simulink model "gm_BlobAnalysisHDL"  (R2022b)
settings: Solver=FixedStepDiscrete  StartTime=0.0  StopTime=1/60  RelTol=1e-3
PreLoadFcn:
  | model_init_cca
InitFcn:
  | model_init_cca
undefined symbols (not defined in the file or in its folder): closenhood, gray, MaxBlobs, numCols, numRows, Rec, rgbmap24, SDTV, Ts
libraries: hdlsllib x37, simulink x21, hdlmdlgenlib x7, visionhdlutilities x5, visionhdlio x2, visiontextngfix x2, visionhdlmorphops x1, visionhdlconversions x1, visionsources x1, visiongeotforms x1
(part 2 of 3)

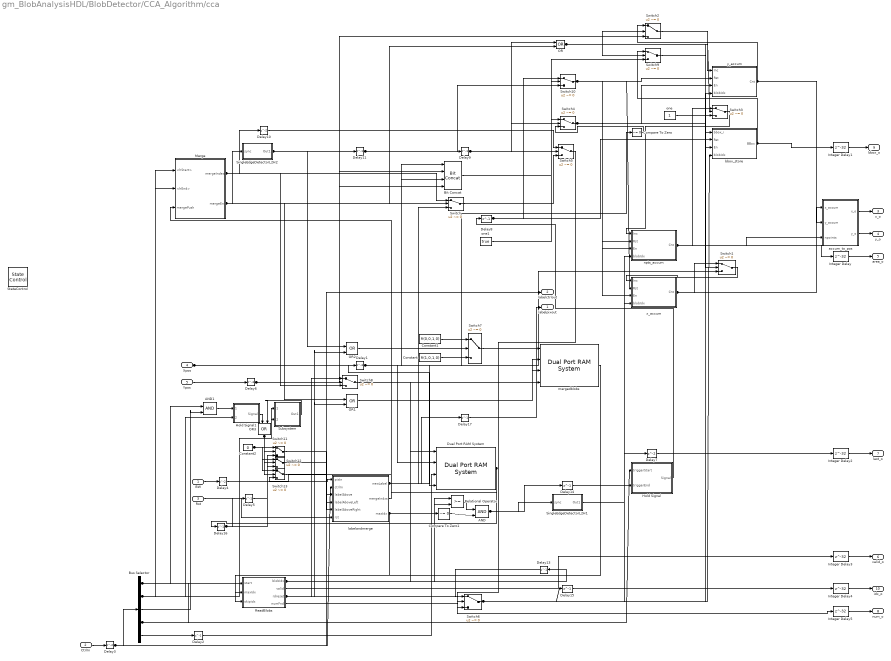
== system gm_BlobAnalysisHDL/BlobDetector/CCA_Algorithm/cca ==
  BW : Inport  OutDataTypeStr=boolean  PortDimensions=1  SampleTime=1.2796101795549e-07
  CtrlIn : Inport  Port=2
  Rst : Inport  Port=3  OutDataTypeStr=boolean  PortDimensions=1  SampleTime=1.2796101795549e-07
  Xpos : Inport  Port=4  OutDataTypeStr=fixdt(0, 9, 0)  PortDimensions=1  SampleTime=1.2796101795549e-07
  Ypos : Inport  Port=5  OutDataTypeStr=uint8  PortDimensions=1  SampleTime=1.2796101795549e-07
  AND : Logic  IconShape=distinctive  AllPortsSameDT=off  OutDataTypeStr=boolean
  AND1 : Logic  IconShape=distinctive  AllPortsSameDT=off  OutDataTypeStr=boolean
  Bit Concat : hdlsllib/Logic and Bit Operations/Bit Concat  numInputs=4
  Bus Selector : BusSelector  OutputSignals=hStart,hEnd,vStart,vEnd,valid
  Compare To Zero : simulink/Logic and Bit Operations/Compare To Zero  relop=~=  OutDataTypeStr=boolean
  Compare To Zero1 : simulink/Logic and Bit Operations/Compare To Zero  relop=~=  OutDataTypeStr=boolean
  Constant : Constant  Value=fi(1,0,1,0)  SampleTime=-1
  Constant1 : Constant  Value=fi(0,0,1,0)  SampleTime=-1
  Constant2 : Constant  Value=0  OutDataTypeStr=fixdt(0,ceil(log2(MaxBlobs)),0)  SampleTime=-1
  Delay1 : Delay  DelayLength=3
  Delay10 : Delay
  Delay{2,5,9,11,13,16..17} (7 alike) : Delay  DelayLength=1
  Delay14 : Delay  DelayLength=1  InitialCondition=0
  Delay15 : Delay  DelayLength=1  InitialCondition=0
  Delay3 : Delay
  Delay4 : Delay
  Delay6 : Delay  DelayLength=3
  Delay7 : Delay  InitialCondition=0
  Delay8 : Delay  DelayLength=1  InitialCondition=0
  Dual Port RAM System : hdlsllib/HDL RAMs/Dual Port RAM System  RAMType=Simple dual port  WriteOutputValue=Old data  RAMInitialValue=0  SimulateUsing=Code generation
  Hold Signal : Subsystem
  Hold Signal1 : Subsystem
  Integer Delay{,1..5} (6 alike) : Delay  DelayLength=32  InitialCondition=0
  Merge : Subsystem
  OR{,1..3} (4 alike) : Logic  Operator=OR  IconShape=distinctive  AllPortsSameDT=off  OutDataTypeStr=boolean
  ReadBlobs : Subsystem
  Relational Operator : RelationalOperator  OutDataTypeStr=boolean  RndMeth=Simplest  InputSameDT=off
  SingleEdgeDetectorL2H1 : Subsystem
  SingleEdgeDetectorL2H2 : Subsystem
  StateControl : StateControl  StateControl=Synchronous
  Subsystem : Subsystem
  Switch{,1..13} (14 alike) : Switch  Criteria=u2 ~= 0  SaturateOnIntegerOverflow=off  InputSameDT=off
  accum_to_pos : Subsystem
  bbox_store : Subsystem  mask(Accumulator){MaxVal=double(76800)}
      mask prompts: MaxVal "Accumulator Maximum Value"
      mask help: Accumulate values
  labelandmerge : Subsystem
  mergedblobs : hdlsllib/HDL RAMs/Dual Port RAM System  RAMType=Simple dual port  WriteOutputValue=Old data  RAMInitialValue=0  SimulateUsing=Code generation
  npts_accum : Subsystem  mask(Accumulator){MaxVal=double(76800)}
      mask prompts: MaxVal "Accumulator Maximum Value"
      mask help: Accumulate values
  one : Constant  OutDataTypeStr=Inherit: Inherit via back propagation  SampleTime=-1
  one1 : Constant  Value=true  OutDataTypeStr=Inherit: Inherit via back propagation  SampleTime=-1
  x_accum : Subsystem  mask(Accumulator){MaxVal=double(12326400)}
      mask prompts: MaxVal "Accumulator Maximum Value"
      mask help: Accumulate values
  y_accum : Subsystem  mask(Accumulator){MaxVal=double(9254400)}
      mask prompts: MaxVal "Accumulator Maximum Value"
      mask help: Accumulate values
  labelpixout : Outport  SampleTime=1.2796101795549e-07  VectorParamsAs1DForOutWhenUnconnected=off
  labelctrlout : Outport  Port=2  VectorParamsAs1DForOutWhenUnconnected=off
  x_o : Outport  Port=3  SampleTime=1.2796101795549e-07  VectorParamsAs1DForOutWhenUnconnected=off
  y_o : Outport  Port=4  SampleTime=1.2796101795549e-07  VectorParamsAs1DForOutWhenUnconnected=off
  area_o : Outport  Port=5  SampleTime=1.2796101795549e-07  VectorParamsAs1DForOutWhenUnconnected=off
  valid_o : Outport  Port=6  SampleTime=1.2796101795549e-07  VectorParamsAs1DForOutWhenUnconnected=off
  last_o : Outport  Port=7  SampleTime=1.2796101795549e-07  VectorParamsAs1DForOutWhenUnconnected=off
  num_o : Outport  Port=8  SampleTime=1.2796101795549e-07  VectorParamsAs1DForOutWhenUnconnected=off
  bbox_o : Outport  Port=9  SampleTime=1.2796101795549e-07  VectorParamsAs1DForOutWhenUnconnected=off
  idx_o : Outport  Port=10  SampleTime=1.2796101795549e-07  VectorParamsAs1DForOutWhenUnconnected=off
  wires:
  AND/1 -> Delay14/1, SingleEdgeDetectorL2H1/1(sync)
  AND1/1 -> Hold Signal1/1(triggerStart)
  Bit Concat/1 -> Switch9/3
  Bus Selector/1 -> AND1/1, Subsystem/1(<hStart>), Merge/1(<hStart>)
  Bus Selector/2 -> Subsystem/2(<hEnd>), Hold Signal1/2(triggerEnd), Merge/2(<hEnd>)
  Bus Selector/3 -> AND1/2
  Bus Selector/4 -> Hold Signal/1(triggerStart), ReadBlobs/1(start)
  Bus Selector/5 -> Delay2/1
  Compare To Zero/1 -> Switch4/3
  Compare To Zero1/1 -> AND/2
  Constant/1 -> Switch7/3
  Constant1/1 -> Switch7/1
  Constant2/1 -> Switch13/1, Switch12/1, Switch11/1
  Delay1/1 -> Bit Concat/3, Bit Concat/1, Switch1/3, Dual Port RAM System/2
  Delay10/1 -> Switch5/1
  Delay11/1 -> Switch10/3, Delay9/1
  Delay13/1 -> Switch6/1
  Delay14/1 -> Hold Signal/2(triggerEnd)
  Delay15/1 -> Integer Delay4/1
  Delay17/1 -> labelpixout/1
  Delay2/1 -> Dual Port RAM System/3
  Delay3/1 -> Bus Selector/1, labelctrlout/1, labelandmerge/2(ctrlIn)
  Delay4/1 -> labelandmerge/1(pixIn)
  Delay6/1 -> Bit Concat/4, Bit Concat/2, Switch2/3
  Delay7/1 -> Integer Delay2/1
  Delay8/1 -> Switch10/2, Switch10/1, bbox_store/2(Rst)
  Delay9/1 -> Switch5/2, Switch4/2, OR/1
  Hold Signal/1(Signal) -> Delay8/1
  Hold Signal1/1(Signal) -> OR3/1
  Integer Delay/1 -> area_o/1
  Integer Delay1/1 -> bbox_o/1
  Integer Delay2/1 -> last_o/1
  Integer Delay3/1 -> valid_o/1
  Integer Delay4/1 -> idx_o/1
  Integer Delay5/1 -> num_o/1
  Merge/1(mergeIndex) -> Switch/1, Delay10/1, Switch8/3
  Merge/2(mergeEn) -> Switch/2, OR/2, SingleEdgeDetectorL2H2/1(sync), OR1/1
  OR/1 -> Switch9/2, Switch1/2, Switch2/2, Switch3/2
  OR3/1 -> Switch13/2, Switch12/2, Switch11/2
  ReadBlobs/1(blobIdx) -> Relational Operator/1, Delay13/1, Switch8/1, mergedblobs/4
  ReadBlobs/2(valid) -> Integer Delay3/1
  ReadBlobs/3(rdreset) -> Switch6/2, Switch8/2, OR2/2, OR1/2
  ReadBlobs/4(numFnd) -> Integer Delay5/1
  Relational Operator/1 -> AND/1
  SingleEdgeDetectorL2H1/1(Out1) -> Delay7/1
  SingleEdgeDetectorL2H2/1(Out1) -> Delay11/1, OR2/1
  Subsystem/1(Out1) -> OR3/2
  Switch/1 -> Switch5/3
  Switch10/1 -> x_accum/2(Rst), y_accum/2(Rst), npts_accum/2(Rst)
  Switch4/1 -> bbox_store/3(En), x_accum/3(En), y_accum/3(En), npts_accum/3(En)
  Switch5/1 -> Switch6/3
  Switch6/1 -> Delay15/1, bbox_store/4(blobIdx), x_accum/4(blobIdx), y_accum/4(blobIdx), npts_accum/4(blobIdx)
  accum_to_pos/1(x_o) -> x_o/1
  accum_to_pos/2(y_o) -> y_o/1
  bbox_store/1(BBox) -> Integer Delay1/1, Switch9/1
  labelandmerge/1(newLabel) -> Switch/3, Compare To Zero/1, Delay17/1, Dual Port RAM System/1
  labelandmerge/2(mergeIndxs) -> Merge/3(mergePush)
  labelandmerge/3(maxIdx) -> Relational Operator/2, Compare To Zero1/1, ReadBlobs/2(maxIdx)
  npts_accum/1(Cnt) -> Integer Delay/1, accum_to_pos/3(npoints), Switch3/1
  one/1 -> Switch3/3
  one1/1 -> Switch4/1
  x_accum/1(Cnt) -> accum_to_pos/1(x_accum), Switch1/1
  y_accum/1(Cnt) -> accum_to_pos/2(y_accum), Switch2/1
  BW/1 -> Delay4/1
  CtrlIn/1 -> Delay3/1
  Rst/1 -> labelandmerge/6(rst)
  Xpos/1 -> Delay1/1, Dual Port RAM System/4
  Ypos/1 -> Delay6/1
  Switch9/1 -> bbox_store/1(bbox_i)
  Switch13/1 -> labelandmerge/5(labelAboveRight)
  Switch12/1 -> labelandmerge/4(labelAboveLeft)
  Delay5/1 -> Switch12/3
  Switch11/1 -> labelandmerge/3(labelAbove)
  Dual Port RAM System/1 -> Switch13/3, Delay16/1
  Delay16/1 -> Switch11/3, Delay5/1
  OR1/1 -> mergedblobs/3
  Switch8/1 -> mergedblobs/2
  Switch7/1 -> mergedblobs/1
  OR2/1 -> Switch7/2
  mergedblobs/1 -> ReadBlobs/3(skipidx)
  Switch1/1 -> x_accum/1(Inc)
  Switch2/1 -> y_accum/1(Inc)
  Switch3/1 -> npts_accum/1(Inc)

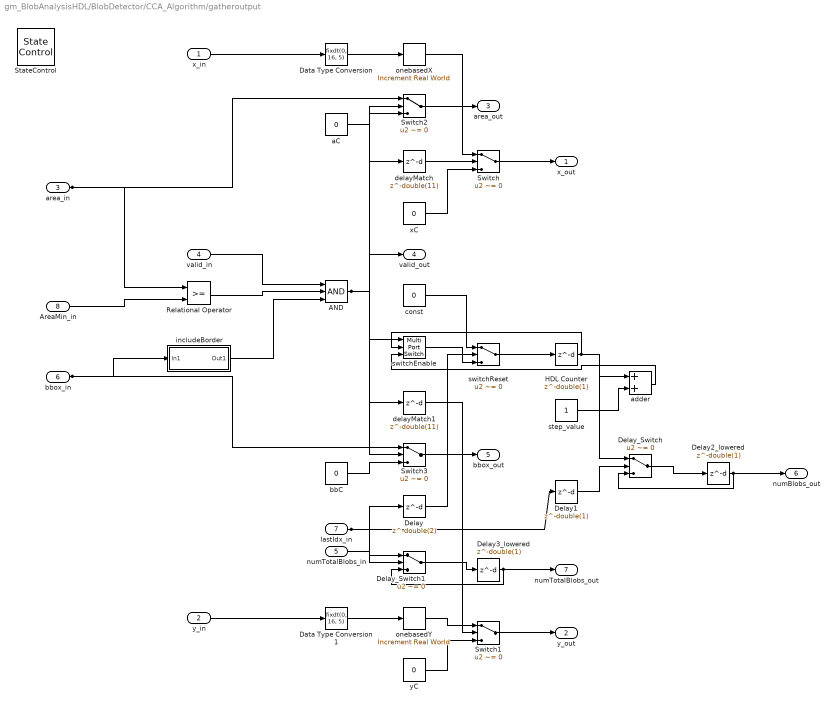
== system gm_BlobAnalysisHDL/BlobDetector/CCA_Algorithm/gatheroutput ==
  x_in : Inport  OutDataTypeStr=fixdt(0, 56, 30)  PortDimensions=1  SampleTime=1.2796101795549e-07
  y_in : Inport  Port=2  OutDataTypeStr=fixdt(0, 56, 30)  PortDimensions=1  SampleTime=1.2796101795549e-07
  area_in : Inport  Port=3  OutDataTypeStr=fixdt(0, 17, 0)  PortDimensions=1  SampleTime=1.2796101795549e-07
  valid_in : Inport  Port=4  OutDataTypeStr=boolean  PortDimensions=1  SampleTime=1.2796101795549e-07
  numTotalBlobs_in : Inport  Port=5  OutDataTypeStr=uint16  PortDimensions=1  SampleTime=1.2796101795549e-07
  bbox_in : Inport  Port=6  OutDataTypeStr=fixdt(0, 34, 0)  PortDimensions=1  SampleTime=1.2796101795549e-07
  lastIdx_in : Inport  Port=7  OutDataTypeStr=boolean  PortDimensions=1  SampleTime=1.2796101795549e-07
  AreaMin_in : Inport  Port=8  OutDataTypeStr=uint32  PortDimensions=1  SampleTime=1.2796101795549e-07
  AND : Logic  Inputs=3  AllPortsSameDT=off  OutDataTypeStr=boolean  SampleTime=1.2796101795549e-07
  Data Type Conversion : DataTypeConversion  OutDataTypeStr=fixdt(0, 16, 5)  SampleTime=1.2796101795549e-07  SaturateOnIntegerOverflow=off  RndMeth=Floor
  Data Type Conversion1 : DataTypeConversion  OutDataTypeStr=fixdt(0, 16, 5)  SampleTime=1.2796101795549e-07  SaturateOnIntegerOverflow=off  RndMeth=Floor
  Delay : Delay  DelayLength=double(2)  InitialCondition=1  SampleTime=1.2796101795549e-07
  Delay1 : Delay  DelayLength=double(1)  InitialCondition=1  SampleTime=1.2796101795549e-07
  Delay2_lowered : Delay  DelayLength=double(1)  InitialCondition=0  SampleTime=1.2796101795549e-07
  Delay3_lowered : Delay  DelayLength=double(1)  InitialCondition=0  SampleTime=1.2796101795549e-07
  Delay_Switch : Switch  Criteria=u2 ~= 0  Threshold=double(0)  OutDataTypeStr=uint16  SampleTime=1.2796101795549e-07  SaturateOnIntegerOverflow=off  InputSameDT=off
  Delay_Switch1 : Switch  Criteria=u2 ~= 0  Threshold=double(0)  OutDataTypeStr=uint16  SampleTime=1.2796101795549e-07  SaturateOnIntegerOverflow=off  InputSameDT=off
  HDL Counter : Delay  DelayLength=double(1)  InitialCondition=0  SampleTime=1.2796101795549e-07
  Relational Operator : RelationalOperator  OutDataTypeStr=boolean  SampleTime=1.2796101795549e-07  InputSameDT=off
  StateControl : StateControl  StateControl=Synchronous
  Switch : Switch  Criteria=u2 ~= 0  Threshold=double(0)  OutDataTypeStr=fixdt(0, 16, 5)  SampleTime=1.2796101795549e-07  SaturateOnIntegerOverflow=off  InputSameDT=off
  Switch1 : Switch  Criteria=u2 ~= 0  Threshold=double(0)  OutDataTypeStr=fixdt(0, 16, 5)  SampleTime=1.2796101795549e-07  SaturateOnIntegerOverflow=off  InputSameDT=off
  Switch2 : Switch  Criteria=u2 ~= 0  Threshold=double(0)  OutDataTypeStr=fixdt(0, 17, 0)  SampleTime=1.2796101795549e-07  SaturateOnIntegerOverflow=off  InputSameDT=off
  Switch3 : Switch  Criteria=u2 ~= 0  Threshold=double(0)  OutDataTypeStr=fixdt(0, 34, 0)  SampleTime=1.2796101795549e-07  SaturateOnIntegerOverflow=off  InputSameDT=off
  aC : Constant  Value=0  OutDataTypeStr=fixdt(0, 17, 0)  SampleTime=1.2796101795549e-07
  adder : Sum  AccumDataTypeStr=uint16  OutDataTypeStr=uint16  SampleTime=1.2796101795549e-07
  bbC : Constant  Value=0  OutDataTypeStr=fixdt(0, 34, 0)  SampleTime=1.2796101795549e-07
  const : Constant  Value=0  VectorParams1D=off  OutDataTypeStr=uint16  SampleTime=1.2796101795549e-07
  delayMatch : Delay  DelayLength=double(11)  InitialCondition=0  SampleTime=1.2796101795549e-07
  delayMatch1 : Delay  DelayLength=double(11)  InitialCondition=0  SampleTime=1.2796101795549e-07
  includeBorder : Subsystem
  onebasedX : simulink/Additional Math & Discrete/Additional Math: Increment - Decrement/Increment Real World
  onebasedY : simulink/Additional Math & Discrete/Additional Math: Increment - Decrement/Increment Real World
  step_value : Constant  VectorParams1D=off  OutDataTypeStr=uint16  SampleTime=1.2796101795549e-07
  switchEnable : MultiPortSwitch  DataPortOrder=Zero-based contiguous  Inputs=2  DiagnosticForDefault=None  zeroidx=on  OutDataTypeStr=uint16  SampleTime=1.2796101795549e-07  SaturateOnIntegerOverflow=off  InputSameDT=off
  switchReset : Switch  Criteria=u2 ~= 0  Threshold=double(0)  OutDataTypeStr=uint16  SampleTime=1.2796101795549e-07  SaturateOnIntegerOverflow=off  InputSameDT=off
  xC : Constant  Value=0  OutDataTypeStr=fixdt(0, 16, 5)  SampleTime=1.2796101795549e-07
  yC : Constant  Value=0  OutDataTypeStr=fixdt(0, 16, 5)  SampleTime=1.2796101795549e-07
  x_out : Outport  SampleTime=1.2796101795549e-07  VectorParamsAs1DForOutWhenUnconnected=off
  y_out : Outport  Port=2  SampleTime=1.2796101795549e-07  VectorParamsAs1DForOutWhenUnconnected=off
  area_out : Outport  Port=3  SampleTime=1.2796101795549e-07  VectorParamsAs1DForOutWhenUnconnected=off
  valid_out : Outport  Port=4  SampleTime=1.2796101795549e-07  VectorParamsAs1DForOutWhenUnconnected=off
  bbox_out : Outport  Port=5  SampleTime=1.2796101795549e-07  VectorParamsAs1DForOutWhenUnconnected=off
  numBlobs_out : Outport  Port=6  SampleTime=1.2796101795549e-07  VectorParamsAs1DForOutWhenUnconnected=off
  numTotalBlobs_out : Outport  Port=7  SampleTime=1.2796101795549e-07  VectorParamsAs1DForOutWhenUnconnected=off
  wires:
  delayMatch/1 -> Switch/2
  Data Type Conversion/1 -> onebasedX/1
  Data Type Conversion1/1 -> onebasedY/1
  Delay/1 -> switchReset/2
  Delay1/1 -> Delay_Switch/2
  Delay2_lowered/1 -> numBlobs_out/1, Delay_Switch/3
  Delay3_lowered/1 -> numTotalBlobs_out/1, Delay_Switch1/3
  Relational Operator/1 -> AND/2
  Switch/1 -> x_out/1
  Switch1/1 -> y_out/1
  Switch2/1 -> area_out/1
  Switch3/1 -> bbox_out/1
  aC/1 -> Switch2/3
  bbC/1 -> Switch3/3
  includeBorder/1(Out1) -> AND/3
  onebasedX/1 -> Switch/1
  onebasedY/1 -> Switch1/1
  xC/1 -> Switch/3
  yC/1 -> Switch1/3
  HDL Counter/1 -> switchEnable/2, adder/1, Delay_Switch/1
  const/1 -> switchReset/1
  step_value/1 -> adder/2
  x_in/1 -> Data Type Conversion/1
  y_in/1 -> Data Type Conversion1/1
  area_in/1 -> Switch2/1, Relational Operator/1
  valid_in/1 -> AND/1
  numTotalBlobs_in/1 -> Delay_Switch1/1
  bbox_in/1 -> Switch3/1, includeBorder/1(In1)
  lastIdx_in/1 -> Delay1/1, Delay/1, Delay_Switch1/2
  AreaMin_in/1 -> Relational Operator/2
  delayMatch1/1 -> Switch1/2
  AND/1 -> delayMatch1/1, delayMatch/1, Switch3/2, Switch2/2, valid_out/1, switchEnable/1
  Delay_Switch1/1 -> Delay3_lowered/1
  adder/1 -> switchEnable/3
  switchEnable/1 -> switchReset/3
  switchReset/1 -> HDL Counter/1
  Delay_Switch/1 -> Delay2_lowered/1

== system gm_BlobAnalysisHDL/BlobDetector/CacheResultForXfer/splitBBox ==
  In1 : Inport  OutDataTypeStr=fixdt(0, 34, 0)  PortDimensions=1  SampleTime=1.2796101795549e-07
  Bit Slice4 : hdlsllib/Logic and Bit Operations/Bit Slice  lidx=ceil(log2(numRows))-1  ridx=0
  Bit Slice5 : hdlsllib/Logic and Bit Operations/Bit Slice  lidx=ceil(log2(numRows))+ceil(log2(numCols))-1  ridx=ceil(log2(numRows))
  Bit Slice6 : hdlsllib/Logic and Bit Operations/Bit Slice  lidx=2*ceil(log2(numRows))+ceil(log2(numCols))-1  ridx=ceil(log2(numRows))+ceil(log2(numCols))
  Bit Slice7 : hdlsllib/Logic and Bit Operations/Bit Slice  lidx=2*ceil(log2(numRows))+2*ceil(log2(numCols))-1  ridx=2*ceil(log2(numRows))+ceil(log2(numCols))
  X1 : Outport  SampleTime=1.2796101795549e-07  VectorParamsAs1DForOutWhenUnconnected=off
  Y1 : Outport  Port=2  SampleTime=1.2796101795549e-07  VectorParamsAs1DForOutWhenUnconnected=off
  X2 : Outport  Port=3  SampleTime=1.2796101795549e-07  VectorParamsAs1DForOutWhenUnconnected=off
  Y2 : Outport  Port=4  SampleTime=1.2796101795549e-07  VectorParamsAs1DForOutWhenUnconnected=off
  wires:
  Bit Slice4/1 -> Y2/1
  Bit Slice5/1 -> X2/1
  Bit Slice6/1 -> Y1/1
  Bit Slice7/1 -> X1/1
  In1/1 -> Bit Slice7/1, Bit Slice6/1, Bit Slice5/1, Bit Slice4/1

== system gm_BlobAnalysisHDL/BlobDetector/CCA_Algorithm/PaletteMap/bit2RGB ==
  In1 : Inport  OutDataTypeStr=fixdt(0, 24, 0)  PortDimensions=1  SampleTime=1.2796101795549e-07
  Blue : simulink/Logic and Bit Operations/Extract Bits  bitsToExtract=Range of bits  numBits=8  bitIdxRange=[0 7]  outScalingMode=Treat bit field as an integer
  Green : simulink/Logic and Bit Operations/Extract Bits  bitsToExtract=Range of bits  numBits=8  bitIdxRange=[8 15]  outScalingMode=Treat bit field as an integer
  Red : simulink/Logic and Bit Operations/Extract Bits  bitsToExtract=Range of bits  numBits=8  bitIdxRange=[16 23]  outScalingMode=Treat bit field as an integer
  Vector Concatenate : Concatenate  NumInputs=3  Mode=Multidimensional array  ConcatenateDimension=2
  Out1 : Outport  SampleTime=1.2796101795549e-07  VectorParamsAs1DForOutWhenUnconnected=off
  wires:
  Blue/1 -> Vector Concatenate/3
  Green/1 -> Vector Concatenate/2
  Red/1 -> Vector Concatenate/1
  Vector Concatenate/1 -> Out1/1
  In1/1 -> Red/1, Green/1, Blue/1

== system gm_BlobAnalysisHDL/BlobDetector/CCA_Algorithm/Pixel Stream FIFO/CastIfBoolean ==
  u : Inport  OutDataTypeStr=uint8  PortDimensions=1  SampleTime=1.2796101795549e-07
  visionhdlutilities_c1_CastIfBoolean : MATLAB Function  TreatAsAtomicUnit=on
      settings: LibrarySourceBlock=visionhdlutilities/Pixel Stream FIFO/CastIfBoolean
  y : Outport  SampleTime=1.2796101795549e-07  VectorParamsAs1DForOutWhenUnconnected=off
  wires:
  visionhdlutilities_c1_CastIfBoolean/1(y) -> y/1
  u/1 -> visionhdlutilities_c1_CastIfBoolean/1(u)

== system gm_BlobAnalysisHDL/BlobDetector/CCA_Algorithm/Pixel Stream FIFO/Input Control Validation  ==
  ctrlIn : Inport
  ControlBalance{,1..6} (7 alike) : Delay  DelayLength=1
  InLineInFrameTest : Subsystem
  Logical Operator{1..6} (6 alike) : Logic  AllPortsSameDT=off  OutDataTypeStr=boolean
  Logical Operator7 : Logic  Operator=OR  AllPortsSameDT=off  OutDataTypeStr=boolean
  Logical Operator8 : Logic  Operator=OR  AllPortsSameDT=off  OutDataTypeStr=boolean
  Pixel Control Bus Creator : visionhdlutilities/Pixel Control Bus Creator
  Pixel Control Bus Selector : BusSelector  OutputSignals=hStart,hEnd,vStart,vEnd,valid
  ctrlOut : Outport  VectorParamsAs1DForOutWhenUnconnected=off
  wires:
  ControlBalance/1 -> Pixel Control Bus Selector/1
  ControlBalance1/1 -> Logical Operator5/1
  ControlBalance2/1 -> Logical Operator6/1, Logical Operator5/2
  ControlBalance3/1 -> Logical Operator3/1
  ControlBalance4/1 -> Logical Operator2/1
  ControlBalance5/1 -> Pixel Control Bus Creator/2
  ControlBalance6/1 -> Pixel Control Bus Creator/4
  InLineInFrameTest/1(InLineInFrame) -> Logical Operator6/2, Logical Operator4/2, Logical Operator3/2, Logical Operator2/2, Logical Operator1/2, ControlBalance1/1
  Logical Operator1/1 -> Logical Operator8/1
  Logical Operator2/1 -> Pixel Control Bus Creator/3
  Logical Operator3/1 -> Pixel Control Bus Creator/1
  Logical Operator4/1 -> Logical Operator8/2, ControlBalance6/1
  Logical Operator5/1 -> Logical Operator7/2
  Logical Operator6/1 -> Logical Operator7/1
  Logical Operator7/1 -> Pixel Control Bus Creator/5
  Logical Operator8/1 -> ControlBalance5/1
  Pixel Control Bus Creator/1 -> ctrlOut/1
  Pixel Control Bus Selector/1 -> ControlBalance3/1
  Pixel Control Bus Selector/2 -> Logical Operator1/1
  Pixel Control Bus Selector/3 -> ControlBalance4/1
  Pixel Control Bus Selector/4 -> Logical Operator4/1
  Pixel Control Bus Selector/5 -> ControlBalance2/1
  ctrlIn/1 -> ControlBalance/1, InLineInFrameTest/1(ctrlIn)

== system gm_BlobAnalysisHDL/BlobDetector/CCA_Algorithm/Pixel Stream FIFO/InputSizeValidation ==
  pixelIn : Inport  OutDataTypeStr=uint8  PortDimensions=1  SampleTime=1.2796101795549e-07
  ctrlIn : Inport  Port=2
  noHDL : visionhdlutilities/Pixel Stream FIFO/InputSizeValidation/noHDL  SystemSampleTime=-1  VariantActivationTime=update diagram  Latency=0  AutoFrameSizeCalculation=off
  wires:
  pixelIn/1 -> noHDL/1
  ctrlIn/1 -> noHDL/2

== system gm_BlobAnalysisHDL/BlobDetector/CCA_Algorithm/Pixel Stream FIFO/Memory Controller ==
  hEnd : Inport  OutDataTypeStr=boolean  PortDimensions=1  SampleTime=1.2796101795549e-07
  readCountIn : Inport  Port=2  OutDataTypeStr=fixdt(0, 11, 0)  PortDimensions=1  SampleTime=1.2796101795549e-07
  writeCountLimit : Inport  Port=3  OutDataTypeStr=fixdt(0, 11, 0)  PortDimensions=1  SampleTime=1.2796101795549e-07
  vStart : Inport  Port=4  OutDataTypeStr=boolean  PortDimensions=1  SampleTime=1.2796101795549e-07
  visionhdlutilities_c2_Memory_Controller : MATLAB Function  TreatAsAtomicUnit=on
      settings: LibrarySourceBlock=visionhdlutilities/Pixel Stream FIFO/Memory Controller
  pop : Outport  SampleTime=1.2796101795549e-07  VectorParamsAs1DForOutWhenUnconnected=off
  wires:
  visionhdlutilities_c2_Memory_Controller/1(pop) -> pop/1
  hEnd/1 -> visionhdlutilities_c2_Memory_Controller/1(hEnd)
  readCountIn/1 -> visionhdlutilities_c2_Memory_Controller/2(readCountIn)
  writeCountLimit/1 -> visionhdlutilities_c2_Memory_Controller/3(writeCountLimit)
  vStart/1 -> visionhdlutilities_c2_Memory_Controller/4(vStart)

== system gm_BlobAnalysisHDL/BlobDetector/CCA_Algorithm/Pixel Stream FIFO/ReshapeFunction ==
  u : Inport  OutDataTypeStr=uint8  PortDimensions=1  SampleTime=1.2796101795549e-07
  v : Inport  Port=2  OutDataTypeStr=uint8  PortDimensions=1  SampleTime=1.2796101795549e-07
  visionhdlutilities_c3_ReshapeFunction : MATLAB Function  TreatAsAtomicUnit=on
      settings: LibrarySourceBlock=visionhdlutilities/Pixel Stream FIFO/ReshapeFunction
  y : Outport  SampleTime=1.2796101795549e-07
  wires:
  visionhdlutilities_c3_ReshapeFunction/1(y) -> y/1
  u/1 -> visionhdlutilities_c3_ReshapeFunction/1(u)
  v/1 -> visionhdlutilities_c3_ReshapeFunction/2(v)

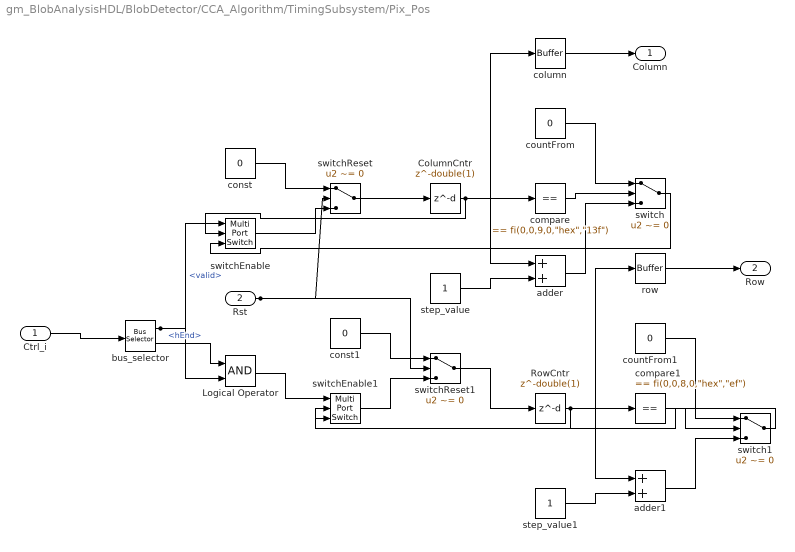
== system gm_BlobAnalysisHDL/BlobDetector/CCA_Algorithm/TimingSubsystem/Pix_Pos ==
  Ctrl_i : Inport
  Rst : Inport  Port=2  OutDataTypeStr=boolean  PortDimensions=1  SampleTime=1.2796101795549e-07
  ColumnCntr : Delay  DelayLength=double(1)  InitialCondition=0  SampleTime=1.2796101795549e-07
  Logical Operator : Logic  AllPortsSameDT=off  OutDataTypeStr=boolean  SampleTime=1.2796101795549e-07
  RowCntr : Delay  DelayLength=double(1)  InitialCondition=0  SampleTime=1.2796101795549e-07
  adder : Sum  AccumDataTypeStr=fixdt(0, 9, 0)  OutDataTypeStr=fixdt(0, 9, 0)  SampleTime=1.2796101795549e-07
  adder1 : Sum  AccumDataTypeStr=uint8  OutDataTypeStr=uint8  SampleTime=1.2796101795549e-07
  bus_selector : BusSelector  OutputSignals=valid,hEnd
  column : hdlmdlgenlib/Buffer
  compare : simulink/Logic and Bit Operations/Compare To Constant  relop===  const="fi(0,0,9,0,\"hex\",\"13f\")"  OutDataTypeStr=boolean
  compare1 : simulink/Logic and Bit Operations/Compare To Constant  relop===  const="fi(0,0,8,0,\"hex\",\"ef\")"  OutDataTypeStr=boolean
  const : Constant  Value=0  VectorParams1D=off  OutDataTypeStr=fixdt(0, 9, 0)  SampleTime=1.2796101795549e-07
  const1 : Constant  Value=0  VectorParams1D=off  OutDataTypeStr=uint8  SampleTime=1.2796101795549e-07
  countFrom : Constant  Value=0  VectorParams1D=off  OutDataTypeStr=fixdt(0, 9, 0)  SampleTime=1.2796101795549e-07
  countFrom1 : Constant  Value=0  VectorParams1D=off  OutDataTypeStr=uint8  SampleTime=1.2796101795549e-07
  row : hdlmdlgenlib/Buffer
  step_value : Constant  VectorParams1D=off  OutDataTypeStr=fixdt(0, 9, 0)  SampleTime=1.2796101795549e-07
  step_value1 : Constant  VectorParams1D=off  OutDataTypeStr=uint8  SampleTime=1.2796101795549e-07
  switch : Switch  Criteria=u2 ~= 0  Threshold=double(0)  OutDataTypeStr=fixdt(0, 9, 0)  SampleTime=1.2796101795549e-07  SaturateOnIntegerOverflow=off  InputSameDT=off
  switch1 : Switch  Criteria=u2 ~= 0  Threshold=double(0)  OutDataTypeStr=uint8  SampleTime=1.2796101795549e-07  SaturateOnIntegerOverflow=off  InputSameDT=off
  switchEnable : MultiPortSwitch  DataPortOrder=Zero-based contiguous  Inputs=2  DiagnosticForDefault=None  zeroidx=on  OutDataTypeStr=fixdt(0, 9, 0)  SampleTime=1.2796101795549e-07  SaturateOnIntegerOverflow=off  InputSameDT=off
  switchEnable1 : MultiPortSwitch  DataPortOrder=Zero-based contiguous  Inputs=2  DiagnosticForDefault=None  zeroidx=on  OutDataTypeStr=uint8  SampleTime=1.2796101795549e-07  SaturateOnIntegerOverflow=off  InputSameDT=off
  switchReset : Switch  Criteria=u2 ~= 0  Threshold=double(0)  OutDataTypeStr=fixdt(0, 9, 0)  SampleTime=1.2796101795549e-07  SaturateOnIntegerOverflow=off  InputSameDT=off
  switchReset1 : Switch  Criteria=u2 ~= 0  Threshold=double(0)  OutDataTypeStr=uint8  SampleTime=1.2796101795549e-07  SaturateOnIntegerOverflow=off  InputSameDT=off
  Column : Outport  SampleTime=1.2796101795549e-07  VectorParamsAs1DForOutWhenUnconnected=off
  Row : Outport  Port=2  SampleTime=1.2796101795549e-07  VectorParamsAs1DForOutWhenUnconnected=off
  wires:
  bus_selector/1 -> Logical Operator/2, switchEnable/1  "<valid>"
  bus_selector/2 -> Logical Operator/1  "<hEnd>"
  column/1 -> Column/1
  Logical Operator/1 -> switchEnable1/1
  row/1 -> Row/1
  ColumnCntr/1 -> column/1, switchEnable/2, compare/1, adder/1
  const/1 -> switchReset/1
  step_value/1 -> adder/2
  countFrom/1 -> switch/1
  RowCntr/1 -> row/1, switchEnable1/2, compare1/1, adder1/1
  const1/1 -> switchReset1/1
  step_value1/1 -> adder1/2
  countFrom1/1 -> switch1/1
  Ctrl_i/1 -> bus_selector/1
  Rst/1 -> switchReset/2, switchReset1/2
  adder/1 -> switch/3
  compare/1 -> switch/2
  switch/1 -> switchEnable/3
  switchEnable/1 -> switchReset/3
  switchReset/1 -> ColumnCntr/1
  adder1/1 -> switch1/3
  compare1/1 -> switch1/2
  switch1/1 -> switchEnable1/3
  switchEnable1/1 -> switchReset1/3
  switchReset1/1 -> RowCntr/1

== system gm_BlobAnalysisHDL/BlobDetector/CCA_Algorithm/TimingSubsystem/create_rst ==
  Video_i : Inport  OutDataTypeStr=boolean  PortDimensions=1  SampleTime=1.2796101795549e-07
  ctrl_i : Inport  Port=2
  Bus Selector : BusSelector  OutputSignals=hStart,vStart,valid
  Delay2 : Delay  DelayLength=1
  Delay3 : Delay  DelayLength=1
  Logical Operator : Logic  Inputs=3  AllPortsSameDT=off  OutDataTypeStr=boolean
  Video_o : Outport  SampleTime=1.2796101795549e-07  VectorParamsAs1DForOutWhenUnconnected=off
  Ctrl_o : Outport  Port=2  VectorParamsAs1DForOutWhenUnconnected=off
  Rst : Outport  Port=3  SampleTime=1.2796101795549e-07  VectorParamsAs1DForOutWhenUnconnected=off
  wires:
  Bus Selector/1 -> Logical Operator/1
  Bus Selector/2 -> Logical Operator/2
  Bus Selector/3 -> Logical Operator/3
  Delay2/1 -> Video_o/1
  Delay3/1 -> Ctrl_o/1
  Logical Operator/1 -> Rst/1
  Video_i/1 -> Delay2/1
  ctrl_i/1 -> Bus Selector/1, Delay3/1

== system gm_BlobAnalysisHDL/BlobDetector/CCA_Algorithm/cca/Hold Signal ==
  triggerStart : Inport  OutDataTypeStr=boolean  PortDimensions=1  SampleTime=1.2796101795549e-07
  triggerEnd : Inport  Port=2  OutDataTypeStr=boolean  PortDimensions=1  SampleTime=1.2796101795549e-07
  Constant5 : Constant  Value=0  OutDataTypeStr=boolean  SampleTime=-1
  Constant6 : Constant  OutDataTypeStr=boolean  SampleTime=-1
  Delay6 : Delay  DelayLength=1  InitialCondition=0  UseCircularBuffer=on
  Logical Operator : Logic  IconShape=distinctive  AllPortsSameDT=off  OutDataTypeStr=boolean
  Logical Operator1 : Logic  Operator=NOT  IconShape=distinctive  AllPortsSameDT=off  OutDataTypeStr=boolean
  Switch3 : Switch  Criteria=u2 ~= 0  SaturateOnIntegerOverflow=off  InputSameDT=off
  Switch4 : Switch  Criteria=u2 ~= 0  SaturateOnIntegerOverflow=off  InputSameDT=off
  Signal : Outport  SampleTime=1.2796101795549e-07  VectorParamsAs1DForOutWhenUnconnected=off
  wires:
  Constant5/1 -> Switch3/1
  Constant6/1 -> Switch4/1
  Logical Operator/1 -> Switch3/2
  Logical Operator1/1 -> Logical Operator/2
  Switch3/1 -> Signal/1, Delay6/1
  triggerStart/1 -> Logical Operator1/1, Switch4/2
  triggerEnd/1 -> Logical Operator/1
  Switch4/1 -> Switch3/3
  Delay6/1 -> Switch4/3

== system gm_BlobAnalysisHDL/BlobDetector/CCA_Algorithm/cca/Hold Signal1 ==
  triggerStart : Inport  OutDataTypeStr=boolean  PortDimensions=1  SampleTime=1.2796101795549e-07
  triggerEnd : Inport  Port=2  OutDataTypeStr=boolean  PortDimensions=1  SampleTime=1.2796101795549e-07
  Constant5 : Constant  Value=0  OutDataTypeStr=boolean  SampleTime=-1
  Constant6 : Constant  OutDataTypeStr=boolean  SampleTime=-1
  Delay6 : Delay  DelayLength=1  InitialCondition=0  UseCircularBuffer=on
  Logical Operator : Logic  IconShape=distinctive  AllPortsSameDT=off  OutDataTypeStr=boolean
  Logical Operator1 : Logic  Operator=NOT  IconShape=distinctive  AllPortsSameDT=off  OutDataTypeStr=boolean
  Switch3 : Switch  Criteria=u2 ~= 0  SaturateOnIntegerOverflow=off  InputSameDT=off
  Switch4 : Switch  Criteria=u2 ~= 0  SaturateOnIntegerOverflow=off  InputSameDT=off
  Signal : Outport  SampleTime=1.2796101795549e-07  VectorParamsAs1DForOutWhenUnconnected=off
  wires:
  Constant5/1 -> Switch3/1
  Constant6/1 -> Switch4/1
  Logical Operator/1 -> Switch3/2
  Logical Operator1/1 -> Logical Operator/2
  Switch3/1 -> Signal/1, Delay6/1
  triggerStart/1 -> Logical Operator1/1, Switch4/2
  triggerEnd/1 -> Logical Operator/1
  Switch4/1 -> Switch3/3
  Delay6/1 -> Switch4/3

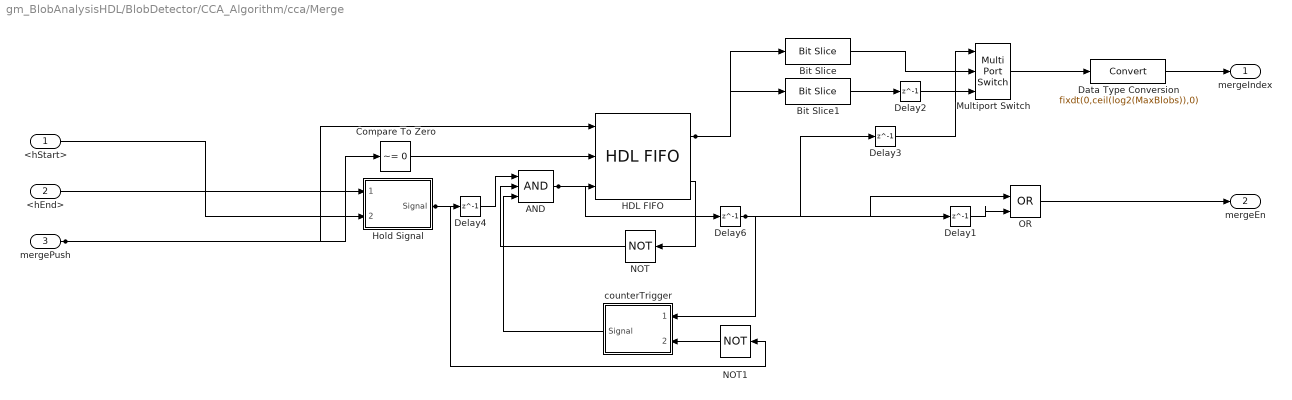
== system gm_BlobAnalysisHDL/BlobDetector/CCA_Algorithm/cca/Merge ==
  <hStart> : Inport  OutDataTypeStr=boolean  PortDimensions=1  SampleTime=1.2796101795549e-07
  <hEnd> : Inport  Port=2  OutDataTypeStr=boolean  PortDimensions=1  SampleTime=1.2796101795549e-07
  mergePush : Inport  Port=3  OutDataTypeStr=uint32  PortDimensions=1  SampleTime=1.2796101795549e-07
  AND : Logic  Inputs=3  IconShape=distinctive  AllPortsSameDT=off  OutDataTypeStr=boolean
  Bit Slice : hdlsllib/Logic and Bit Operations/Bit Slice  lidx=15  ridx=0
  Bit Slice1 : hdlsllib/Logic and Bit Operations/Bit Slice  lidx=31  ridx=16
  Compare To Zero : simulink/Logic and Bit Operations/Compare To Zero  relop=~=  OutDataTypeStr=boolean
  Data Type Conversion : DataTypeConversion  OutDataTypeStr=fixdt(0,ceil(log2(MaxBlobs)),0)  SaturateOnIntegerOverflow=off  RndMeth=Floor
  Delay{1..4,6} (5 alike) : Delay  DelayLength=1
  HDL FIFO : hdlsllib/HDL RAMs/HDL FIFO  fifo_size=100  mode=Classic  ratio=1  push_msg=Warning  pop_msg=Warning  show_empty=on  show_full=off  show_num=off  LabelModeActiveChoice_Mode=Classic  rst_port=off
  Hold Signal : Subsystem
  Multiport Switch : MultiPortSwitch  DataPortOrder=Zero-based contiguous  Inputs=2  DiagnosticForDefault=None  zeroidx=on  SaturateOnIntegerOverflow=off  InputSameDT=off
  NOT : Logic  Operator=NOT  IconShape=distinctive  AllPortsSameDT=off  OutDataTypeStr=boolean
  NOT1 : Logic  Operator=NOT  IconShape=distinctive  AllPortsSameDT=off  OutDataTypeStr=boolean
  OR : Logic  Operator=OR  IconShape=distinctive  AllPortsSameDT=off  OutDataTypeStr=boolean
  counterTrigger : Subsystem  mask{cntValue=double(3)}
      mask prompts: cntValue "Count To Value"
  mergeIndex : Outport  SampleTime=1.2796101795549e-07  VectorParamsAs1DForOutWhenUnconnected=off
  mergeEn : Outport  Port=2  SampleTime=1.2796101795549e-07  VectorParamsAs1DForOutWhenUnconnected=off
  wires:
  Bit Slice/1 -> Multiport Switch/2
  Bit Slice1/1 -> Delay2/1
  Compare To Zero/1 -> HDL FIFO/2
  Data Type Conversion/1 -> mergeIndex/1
  Delay1/1 -> OR/2
  Delay2/1 -> Multiport Switch/3
  Delay3/1 -> Multiport Switch/1
  Delay4/1 -> AND/1
  Delay6/1 -> OR/1, Delay3/1, Delay1/1, counterTrigger/1(triggerStart)
  HDL FIFO/1 -> Bit Slice1/1, Bit Slice/1
  Hold Signal/1(Signal) -> NOT1/1, Delay4/1
  Multiport Switch/1 -> Data Type Conversion/1
  NOT1/1 -> counterTrigger/2(suppress)
  OR/1 -> mergeEn/1
  <hStart>/1 -> Hold Signal/2(triggerEnd)
  <hEnd>/1 -> Hold Signal/1(triggerStart)
  mergePush/1 -> Compare To Zero/1, HDL FIFO/1
  counterTrigger/1(Signal) -> AND/3
  NOT/1 -> AND/2
  AND/1 -> Delay6/1, HDL FIFO/3
  HDL FIFO/2 -> NOT/1

== system gm_BlobAnalysisHDL/BlobDetector/CCA_Algorithm/cca/ReadBlobs ==
  start : Inport  OutDataTypeStr=boolean  PortDimensions=1  SampleTime=1.2796101795549e-07
  maxIdx : Inport  Port=2  OutDataTypeStr=fixdt(0, 11, 0)  PortDimensions=1  SampleTime=1.2796101795549e-07
  skipidx : Inport  Port=3  OutDataTypeStr=fixdt(0, 1, 0)  PortDimensions=1  SampleTime=1.2796101795549e-07
  ReadBlobs : MATLAB Function  TreatAsAtomicUnit=on
  blobIdx : Outport  SampleTime=1.2796101795549e-07  VectorParamsAs1DForOutWhenUnconnected=off
  valid : Outport  Port=2  SampleTime=1.2796101795549e-07  VectorParamsAs1DForOutWhenUnconnected=off
  rdreset : Outport  Port=3  SampleTime=1.2796101795549e-07  VectorParamsAs1DForOutWhenUnconnected=off
  numFnd : Outport  Port=4  SampleTime=1.2796101795549e-07  VectorParamsAs1DForOutWhenUnconnected=off
  wires:
  ReadBlobs/1(blobIdx) -> blobIdx/1
  ReadBlobs/2(valid) -> valid/1
  ReadBlobs/3(rdreset) -> rdreset/1
  ReadBlobs/4(numFnd) -> numFnd/1
  start/1 -> ReadBlobs/1(start)
  maxIdx/1 -> ReadBlobs/2(maxIdx)
  skipidx/1 -> ReadBlobs/3(skipidx)

== system gm_BlobAnalysisHDL/BlobDetector/CCA_Algorithm/cca/SingleEdgeDetectorL2H1 ==
  sync : Inport  OutDataTypeStr=boolean  PortDimensions=1  SampleTime=1.2796101795549e-07
  Logical Operator : Logic  Operator=XOR  IconShape=distinctive  AllPortsSameDT=off  OutDataTypeStr=boolean
  Logical Operator2 : Logic  IconShape=distinctive  AllPortsSameDT=off  OutDataTypeStr=boolean
  Unit Delay : UnitDelay  SampleTime=-1  HasFrameUpgradeWarning=on
  Out1 : Outport  SampleTime=1.2796101795549e-07  VectorParamsAs1DForOutWhenUnconnected=off
  wires:
  Logical Operator/1 -> Logical Operator2/1
  Logical Operator2/1 -> Out1/1
  Unit Delay/1 -> Logical Operator/1
  sync/1 -> Logical Operator2/2, Logical Operator/2, Unit Delay/1

== system gm_BlobAnalysisHDL/BlobDetector/CCA_Algorithm/cca/SingleEdgeDetectorL2H2 ==
  sync : Inport  OutDataTypeStr=boolean  PortDimensions=1  SampleTime=1.2796101795549e-07
  Logical Operator : Logic  Operator=XOR  IconShape=distinctive  AllPortsSameDT=off  OutDataTypeStr=boolean
  Logical Operator2 : Logic  IconShape=distinctive  AllPortsSameDT=off  OutDataTypeStr=boolean
  Unit Delay : UnitDelay  SampleTime=-1  HasFrameUpgradeWarning=on
  Out1 : Outport  SampleTime=1.2796101795549e-07  VectorParamsAs1DForOutWhenUnconnected=off
  wires:
  sync/1 -> Unit Delay/1, Logical Operator/2, Logical Operator2/2
  Unit Delay/1 -> Logical Operator/1
  Logical Operator2/1 -> Out1/1
  Logical Operator/1 -> Logical Operator2/1

== system gm_BlobAnalysisHDL/BlobDetector/CCA_Algorithm/cca/Subsystem ==
  <hStart> : Inport  OutDataTypeStr=boolean  PortDimensions=1  SampleTime=1.2796101795549e-07
  <hEnd> : Inport  Port=2  OutDataTypeStr=boolean  PortDimensions=1  SampleTime=1.2796101795549e-07
  Delay{,1..7} (8 alike) : Delay  DelayLength=1  InitialCondition=0  UseCircularBuffer=on
  OR2 : Logic  Operator=OR  Inputs=4  IconShape=distinctive  AllPortsSameDT=off  OutDataTypeStr=boolean
  OR3 : Logic  Operator=OR  Inputs=5  IconShape=distinctive  AllPortsSameDT=off  OutDataTypeStr=boolean
  OR6 : Logic  Operator=OR  IconShape=distinctive  AllPortsSameDT=off  OutDataTypeStr=boolean
  Out1 : Outport  SampleTime=1.2796101795549e-07
  wires:
  Delay/1 -> OR2/2, Delay1/1
  Delay1/1 -> Delay2/1
  Delay2/1 -> OR2/4, Delay3/1
  Delay3/1 -> OR2/3
  Delay4/1 -> OR3/2, Delay5/1
  Delay5/1 -> OR3/3, Delay6/1
  Delay6/1 -> OR3/4, Delay7/1
  Delay7/1 -> OR3/5
  OR2/1 -> OR6/1
  OR3/1 -> OR6/2
  OR6/1 -> Out1/1
  <hStart>/1 -> OR2/1, Delay/1
  <hEnd>/1 -> OR3/1, Delay4/1

== system gm_BlobAnalysisHDL/BlobDetector/CCA_Algorithm/cca/accum_to_pos ==
  x_accum : Inport  OutDataTypeStr=fixdt(0, 24, 0)  PortDimensions=1  SampleTime=1.2796101795549e-07
  y_accum : Inport  Port=2  OutDataTypeStr=fixdt(0, 24, 0)  PortDimensions=1  SampleTime=1.2796101795549e-07
  npoints : Inport  Port=3  OutDataTypeStr=fixdt(0, 17, 0)  PortDimensions=1  SampleTime=1.2796101795549e-07
  Data Type Conversion2 : Subsystem
      mask Display: disp('NFP\nconv');
  Data Type Conversion2_outbuff : hdlmdlgenlib/Buffer
  Data Type Conversion3 : Subsystem
      mask Display: disp('NFP\nconv');
  Data Type Conversion3_outbuff : hdlmdlgenlib/Buffer
  Integer Delay2 : Delay  DelayLength=double(1)  InitialCondition=0  SampleTime=1.2796101795549e-07
  Integer Delay3 : Delay  DelayLength=double(1)  InitialCondition=0  SampleTime=1.2796101795549e-07
  Integer Delay6 : Delay  DelayLength=double(28)  InitialCondition=0  SampleTime=1.2796101795549e-07
  Integer Delay7 : Delay  DelayLength=double(28)  InitialCondition=0  SampleTime=1.2796101795549e-07
  Math Reciprocal1 : Subsystem
      mask Display: disp('NFP\nmath');
  Math Reciprocal1_outbuff : hdlmdlgenlib/Buffer
  delayMatch : Delay  DelayLength=double(14)  InitialCondition=0  SampleTime=1.2796101795549e-07
  delayMatch1 : Delay  DelayLength=double(14)  InitialCondition=0  SampleTime=1.2796101795549e-07
  x_pos : Product  Inputs=**  OutDataTypeStr=fixdt(0, 56, 30)  SampleTime=1.2796101795549e-07
  y_pos : Product  Inputs=**  OutDataTypeStr=fixdt(0, 56, 30)  SampleTime=1.2796101795549e-07
  x_o : Outport  SampleTime=1.2796101795549e-07  VectorParamsAs1DForOutWhenUnconnected=off
  y_o : Outport  Port=2  SampleTime=1.2796101795549e-07  VectorParamsAs1DForOutWhenUnconnected=off
  wires:
  Data Type Conversion3_outbuff/1 -> Math Reciprocal1/1(In1)
  x_pos/1 -> x_o/1
  y_pos/1 -> y_o/1
  delayMatch/1 -> x_pos/1
  delayMatch1/1 -> y_pos/1
  Data Type Conversion2_outbuff/1 -> y_pos/2, x_pos/2
  Integer Delay6/1 -> Integer Delay3/1
  Integer Delay7/1 -> Integer Delay2/1
  Math Reciprocal1_outbuff/1 -> Data Type Conversion2/1(In1)
  Data Type Conversion2/1(Out1) -> Data Type Conversion2_outbuff/1
  Data Type Conversion3/1(Out1) -> Data Type Conversion3_outbuff/1
  Math Reciprocal1/1(Out1) -> Math Reciprocal1_outbuff/1
  Integer Delay2/1 -> delayMatch/1
  Integer Delay3/1 -> delayMatch1/1
  x_accum/1 -> Integer Delay7/1
  y_accum/1 -> Integer Delay6/1
  npoints/1 -> Data Type Conversion3/1(In1)

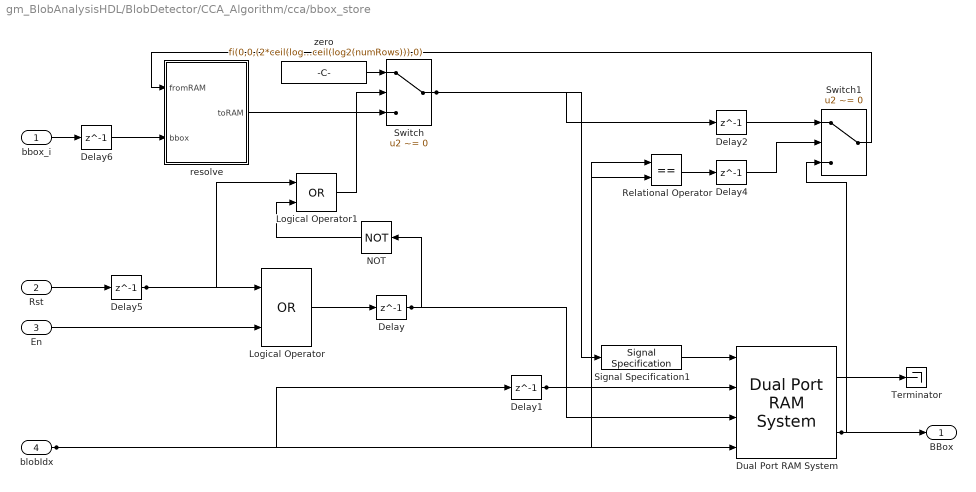
== system gm_BlobAnalysisHDL/BlobDetector/CCA_Algorithm/cca/bbox_store ==
  bbox_i : Inport  OutDataTypeStr=fixdt(0, 34, 0)  PortDimensions=1  SampleTime=1.2796101795549e-07
  Rst : Inport  Port=2  OutDataTypeStr=boolean  PortDimensions=1  SampleTime=1.2796101795549e-07
  En : Inport  Port=3  OutDataTypeStr=boolean  PortDimensions=1  SampleTime=1.2796101795549e-07
  blobIdx : Inport  Port=4  OutDataTypeStr=fixdt(0, 10, 0)  PortDimensions=1  SampleTime=1.2796101795549e-07
  Delay{,1..2,4..6} (6 alike) : Delay  DelayLength=1  InitialCondition=0
  Dual Port RAM System : hdlsllib/HDL RAMs/Dual Port RAM System  RAMType=Dual port  WriteOutputValue=Old data  RAMInitialValue=0  SimulateUsing=Code generation
  Logical Operator : Logic  Operator=OR  IconShape=distinctive  AllPortsSameDT=off  OutDataTypeStr=boolean
  Logical Operator1 : Logic  Operator=OR  IconShape=distinctive  AllPortsSameDT=off  OutDataTypeStr=boolean
  NOT : Logic  Operator=NOT  IconShape=distinctive  AllPortsSameDT=off  OutDataTypeStr=boolean
  Relational Operator : RelationalOperator  Operator===  OutDataTypeStr=boolean  RndMeth=Simplest  InputSameDT=off
  Signal Specification1 : SignalSpecification  OutDataTypeStr=fixdt(0,(2*ceil(log2(numCols))+2*ceil(log2(numRows))),0)
  Switch : Switch  Criteria=u2 ~= 0  OutDataTypeStr=Inherit: Inherit via back propagation  SaturateOnIntegerOverflow=off  InputSameDT=off
  Switch1 : Switch  Criteria=u2 ~= 0  OutDataTypeStr=Inherit: Inherit via back propagation  SaturateOnIntegerOverflow=off  InputSameDT=off
  Terminator : Terminator
  resolve : Subsystem
  zero : Constant  Value=fi(0,0,(2*ceil(log2(numCols))+2*ceil(log2(numRows))),0)  SampleTime=-1
  BBox : Outport  SampleTime=1.2796101795549e-07  VectorParamsAs1DForOutWhenUnconnected=off
  wires:
  Delay/1 -> NOT/1, Dual Port RAM System/3
  Delay1/1 -> Relational Operator/1, Dual Port RAM System/2
  Delay4/1 -> Switch1/2
  Delay5/1 -> Logical Operator1/1, Logical Operator/1
  Delay6/1 -> resolve/2(bbox)
  Dual Port RAM System/1 -> Terminator/1
  Dual Port RAM System/2 -> BBox/1, Switch1/3
  Logical Operator/1 -> Delay/1
  Logical Operator1/1 -> Switch/2
  NOT/1 -> Logical Operator1/2
  Relational Operator/1 -> Delay4/1
  zero/1 -> Switch/1
  bbox_i/1 -> Delay6/1
  Rst/1 -> Delay5/1
  En/1 -> Logical Operator/2
  blobIdx/1 -> Relational Operator/2, Delay1/1, Dual Port RAM System/4
  Signal Specification1/1 -> Dual Port RAM System/1
  Switch1/1 -> resolve/1(fromRAM)
  Switch/1 -> Signal Specification1/1, Delay2/1
  Delay2/1 -> Switch1/1
  resolve/1(toRAM) -> Switch/3

== system gm_BlobAnalysisHDL/BlobDetector/CCA_Algorithm/cca/labelandmerge ==
  pixIn : Inport  OutDataTypeStr=boolean  PortDimensions=1  SampleTime=1.2796101795549e-07
  ctrlIn : Inport  Port=2
  labelAbove : Inport  Port=3  OutDataTypeStr=fixdt(0, 10, 0)  PortDimensions=1  SampleTime=1.2796101795549e-07
  labelAboveLeft : Inport  Port=4  OutDataTypeStr=fixdt(0, 10, 0)  PortDimensions=1  SampleTime=1.2796101795549e-07
  labelAboveRight : Inport  Port=5  OutDataTypeStr=fixdt(0, 10, 0)  PortDimensions=1  SampleTime=1.2796101795549e-07
  rst : Inport  Port=6  OutDataTypeStr=boolean  PortDimensions=1  SampleTime=1.2796101795549e-07
  labelandmerge : MATLAB Function  TreatAsAtomicUnit=on
  newLabel : Outport  SampleTime=1.2796101795549e-07  VectorParamsAs1DForOutWhenUnconnected=off
  mergeIndxs : Outport  Port=2  SampleTime=1.2796101795549e-07  VectorParamsAs1DForOutWhenUnconnected=off
  maxIdx : Outport  Port=3  SampleTime=1.2796101795549e-07  VectorParamsAs1DForOutWhenUnconnected=off
  wires:
  labelandmerge/1(newLabel) -> newLabel/1
  labelandmerge/2(mergeIndxs) -> mergeIndxs/1
  labelandmerge/3(maxIdx) -> maxIdx/1
  pixIn/1 -> labelandmerge/1(pixIn)
  ctrlIn/1 -> labelandmerge/2(ctrlIn)
  labelAbove/1 -> labelandmerge/3(labelAbove)
  labelAboveLeft/1 -> labelandmerge/4(labelAboveLeft)
  labelAboveRight/1 -> labelandmerge/5(labelAboveRight)
  rst/1 -> labelandmerge/6(rst)

== system gm_BlobAnalysisHDL/BlobDetector/CCA_Algorithm/cca/npts_accum ==
  Inc : Inport  OutDataTypeStr=fixdt(0, 17, 0)  PortDimensions=1  SampleTime=1.2796101795549e-07
  Rst : Inport  Port=2  OutDataTypeStr=boolean  PortDimensions=1  SampleTime=1.2796101795549e-07
  En : Inport  Port=3  OutDataTypeStr=boolean  PortDimensions=1  SampleTime=1.2796101795549e-07
  blobIdx : Inport  Port=4  OutDataTypeStr=fixdt(0, 10, 0)  PortDimensions=1  SampleTime=1.2796101795549e-07
  Add : Sum  RndMeth=Zero  SaturateOnIntegerOverflow=on
  Delay{1..6} (6 alike) : Delay  DelayLength=1  InitialCondition=0
  Dual Port RAM System : hdlsllib/HDL RAMs/Dual Port RAM System  RAMType=Dual port  WriteOutputValue=Old data  RAMInitialValue=0  SimulateUsing=Code generation
  Logical Operator : Logic  Operator=OR  IconShape=distinctive  AllPortsSameDT=off  OutDataTypeStr=boolean
  Logical Operator1 : Logic  Operator=OR  IconShape=distinctive  AllPortsSameDT=off  OutDataTypeStr=boolean
  NOT : Logic  Operator=NOT  IconShape=distinctive  AllPortsSameDT=off  OutDataTypeStr=boolean
  Relational Operator : RelationalOperator  Operator===  OutDataTypeStr=boolean  RndMeth=Simplest  InputSameDT=off
  Signal Specification1 : SignalSpecification  OutDataTypeStr=fixdt(0,ceil(log2(MaxVal)),0)
  Switch : Switch  Criteria=u2 ~= 0  OutDataTypeStr=Inherit: Inherit via back propagation  SaturateOnIntegerOverflow=off  InputSameDT=off
  Switch1 : Switch  Criteria=u2 ~= 0  OutDataTypeStr=Inherit: Inherit via back propagation  SaturateOnIntegerOverflow=off  InputSameDT=off
  Terminator : Terminator
  zero : Constant  Value=fi(0,0,ceil(log2(MaxVal)),0)  SampleTime=-1
  Cnt : Outport  SampleTime=1.2796101795549e-07  VectorParamsAs1DForOutWhenUnconnected=off
  wires:
  Delay1/1 -> Relational Operator/1, Dual Port RAM System/2
  Delay3/1 -> Add/2
  Delay4/1 -> Switch1/2
  Delay5/1 -> Logical Operator1/1, Logical Operator/1
  Delay6/1 -> Logical Operator/2
  Dual Port RAM System/1 -> Terminator/1
  Dual Port RAM System/2 -> Cnt/1, Switch1/3
  Logical Operator/1 -> NOT/1, Dual Port RAM System/3
  Logical Operator1/1 -> Switch/2
  NOT/1 -> Logical Operator1/2
  Relational Operator/1 -> Delay4/1
  zero/1 -> Switch/1
  Inc/1 -> Delay3/1
  Rst/1 -> Delay5/1
  En/1 -> Delay6/1
  blobIdx/1 -> Relational Operator/2, Delay1/1, Dual Port RAM System/4
  Signal Specification1/1 -> Dual Port RAM System/1
  Switch1/1 -> Add/1
  Add/1 -> Switch/3
  Switch/1 -> Signal Specification1/1, Delay2/1
  Delay2/1 -> Switch1/1

== system gm_BlobAnalysisHDL/BlobDetector/CCA_Algorithm/cca/x_accum ==
  Inc : Inport  OutDataTypeStr=fixdt(0, 24, 0)  PortDimensions=1  SampleTime=1.2796101795549e-07
  Rst : Inport  Port=2  OutDataTypeStr=boolean  PortDimensions=1  SampleTime=1.2796101795549e-07
  En : Inport  Port=3  OutDataTypeStr=boolean  PortDimensions=1  SampleTime=1.2796101795549e-07
  blobIdx : Inport  Port=4  OutDataTypeStr=fixdt(0, 10, 0)  PortDimensions=1  SampleTime=1.2796101795549e-07
  Add : Sum  RndMeth=Zero  SaturateOnIntegerOverflow=on
  Delay{1..6} (6 alike) : Delay  DelayLength=1  InitialCondition=0
  Dual Port RAM System : hdlsllib/HDL RAMs/Dual Port RAM System  RAMType=Dual port  WriteOutputValue=Old data  RAMInitialValue=0  SimulateUsing=Code generation
  Logical Operator : Logic  Operator=OR  IconShape=distinctive  AllPortsSameDT=off  OutDataTypeStr=boolean
  Logical Operator1 : Logic  Operator=OR  IconShape=distinctive  AllPortsSameDT=off  OutDataTypeStr=boolean
  NOT : Logic  Operator=NOT  IconShape=distinctive  AllPortsSameDT=off  OutDataTypeStr=boolean
  Relational Operator : RelationalOperator  Operator===  OutDataTypeStr=boolean  RndMeth=Simplest  InputSameDT=off
  Signal Specification1 : SignalSpecification  OutDataTypeStr=fixdt(0,ceil(log2(MaxVal)),0)
  Switch : Switch  Criteria=u2 ~= 0  OutDataTypeStr=Inherit: Inherit via back propagation  SaturateOnIntegerOverflow=off  InputSameDT=off
  Switch1 : Switch  Criteria=u2 ~= 0  OutDataTypeStr=Inherit: Inherit via back propagation  SaturateOnIntegerOverflow=off  InputSameDT=off
  Terminator : Terminator
  zero : Constant  Value=fi(0,0,ceil(log2(MaxVal)),0)  SampleTime=-1
  Cnt : Outport  SampleTime=1.2796101795549e-07  VectorParamsAs1DForOutWhenUnconnected=off
  wires:
  Delay1/1 -> Relational Operator/1, Dual Port RAM System/2
  Delay3/1 -> Add/2
  Delay4/1 -> Switch1/2
  Delay5/1 -> Logical Operator1/1, Logical Operator/1
  Delay6/1 -> Logical Operator/2
  Dual Port RAM System/1 -> Terminator/1
  Dual Port RAM System/2 -> Cnt/1, Switch1/3
  Logical Operator/1 -> NOT/1, Dual Port RAM System/3
  Logical Operator1/1 -> Switch/2
  NOT/1 -> Logical Operator1/2
  Relational Operator/1 -> Delay4/1
  zero/1 -> Switch/1
  Inc/1 -> Delay3/1
  Rst/1 -> Delay5/1
  En/1 -> Delay6/1
  blobIdx/1 -> Relational Operator/2, Delay1/1, Dual Port RAM System/4
  Signal Specification1/1 -> Dual Port RAM System/1
  Switch1/1 -> Add/1
  Add/1 -> Switch/3
  Switch/1 -> Signal Specification1/1, Delay2/1
  Delay2/1 -> Switch1/1

== system gm_BlobAnalysisHDL/BlobDetector/CCA_Algorithm/cca/y_accum ==
  Inc : Inport  OutDataTypeStr=fixdt(0, 24, 0)  PortDimensions=1  SampleTime=1.2796101795549e-07
  Rst : Inport  Port=2  OutDataTypeStr=boolean  PortDimensions=1  SampleTime=1.2796101795549e-07
  En : Inport  Port=3  OutDataTypeStr=boolean  PortDimensions=1  SampleTime=1.2796101795549e-07
  blobIdx : Inport  Port=4  OutDataTypeStr=fixdt(0, 10, 0)  PortDimensions=1  SampleTime=1.2796101795549e-07
  Add : Sum  RndMeth=Zero  SaturateOnIntegerOverflow=on
  Delay{,1..5} (6 alike) : Delay  DelayLength=1  InitialCondition=0
  Dual Port RAM System : hdlsllib/HDL RAMs/Dual Port RAM System  RAMType=Dual port  WriteOutputValue=Old data  RAMInitialValue=0  SimulateUsing=Code generation
  Logical Operator : Logic  Operator=OR  IconShape=distinctive  AllPortsSameDT=off  OutDataTypeStr=boolean
  Logical Operator1 : Logic  Operator=OR  IconShape=distinctive  AllPortsSameDT=off  OutDataTypeStr=boolean
  NOT : Logic  Operator=NOT  IconShape=distinctive  AllPortsSameDT=off  OutDataTypeStr=boolean
  Relational Operator : RelationalOperator  Operator===  OutDataTypeStr=boolean  RndMeth=Simplest  InputSameDT=off
  Signal Specification1 : SignalSpecification  OutDataTypeStr=fixdt(0,ceil(log2(MaxVal)),0)
  Switch : Switch  Criteria=u2 ~= 0  OutDataTypeStr=Inherit: Inherit via back propagation  SaturateOnIntegerOverflow=off  InputSameDT=off
  Switch1 : Switch  Criteria=u2 ~= 0  OutDataTypeStr=Inherit: Inherit via back propagation  SaturateOnIntegerOverflow=off  InputSameDT=off
  Terminator : Terminator
  zero : Constant  Value=fi(0,0,ceil(log2(MaxVal)),0)  SampleTime=Ts
  Cnt : Outport  SampleTime=1.2796101795549e-07  VectorParamsAs1DForOutWhenUnconnected=off
  wires:
  Delay/1 -> Logical Operator/2
  Delay1/1 -> Relational Operator/1, Dual Port RAM System/2
  Delay3/1 -> Add/2
  Delay4/1 -> Switch1/2
  Delay5/1 -> Logical Operator1/1, Logical Operator/1
  Dual Port RAM System/1 -> Terminator/1
  Dual Port RAM System/2 -> Cnt/1, Switch1/3
  Logical Operator/1 -> NOT/1, Dual Port RAM System/3
  Logical Operator1/1 -> Switch/2
  NOT/1 -> Logical Operator1/2
  Relational Operator/1 -> Delay4/1
  zero/1 -> Switch/1
  Inc/1 -> Delay3/1
  Rst/1 -> Delay5/1
  En/1 -> Delay/1
  blobIdx/1 -> Relational Operator/2, Delay1/1, Dual Port RAM System/4
  Signal Specification1/1 -> Dual Port RAM System/1
  Switch1/1 -> Add/1
  Add/1 -> Switch/3
  Switch/1 -> Signal Specification1/1, Delay2/1
  Delay2/1 -> Switch1/1

== system gm_BlobAnalysisHDL/BlobDetector/CCA_Algorithm/gatheroutput/includeBorder ==
  In1 : Inport  OutDataTypeStr=fixdt(0, 34, 0)  PortDimensions=1  SampleTime=1.2796101795549e-07
  Out1 : Outport  SampleTime=1.2796101795549e-07  VectorParamsAs1DForOutWhenUnconnected=off
  wires:
  In1/1 -> Out1/1
